simulink model "main_model"  (R2025b)
settings: Solver=VariableStepAuto  StartTime=0.0  StopTime=30  RelTol=1e-3
undefined symbols (not defined in the file or in its folder): A, a, B, C, c, flow_coeff, H, R, W
settings Model: Creator=janek  LastModifiedBy=janek

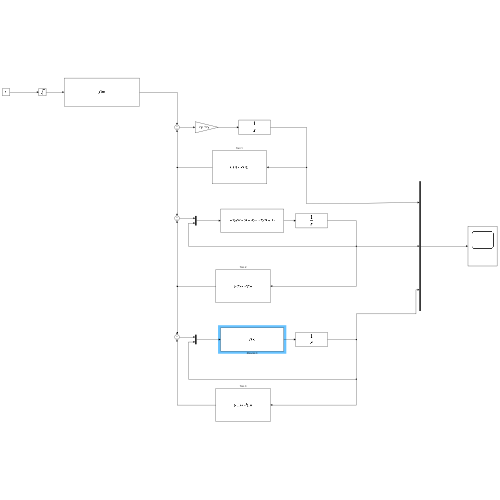
[thumbnail: Simulink's stored preview of the top-level diagram]
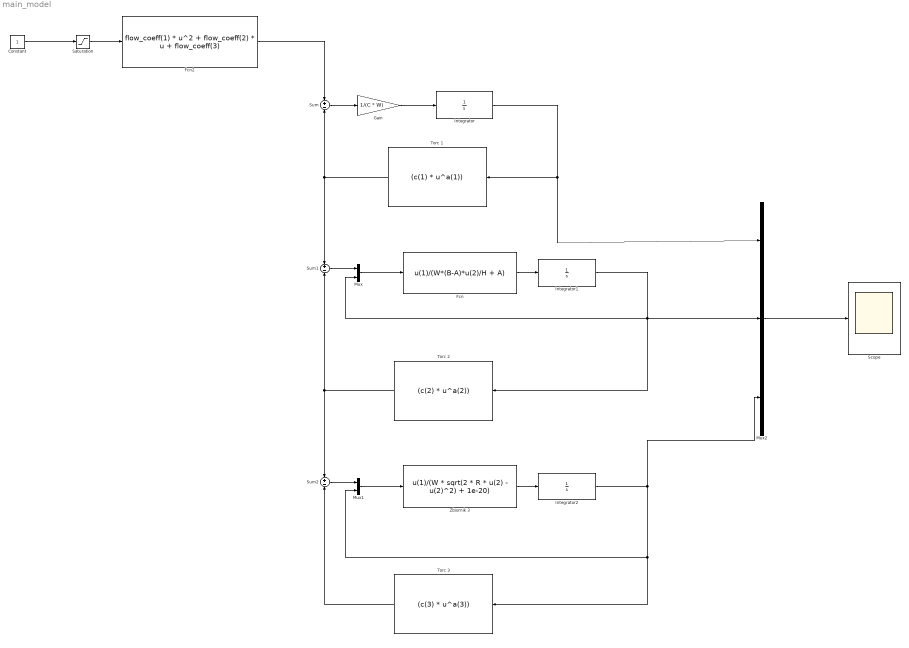
== system main_model ==
  Constant : Constant
  Fcn : Fcn  Expr=u(1)/(W*(B-A)*u(2)/H + A)
  Fcn2 : Fcn  Expr=flow_coeff(1) * u^2 + flow_coeff(2) * u + flow_coeff(3)
  Gain : Gain  Gain=1/(C * W)
  Integrator : Integrator
  Integrator1 : Integrator
  Integrator2 : Integrator
  Mux : Mux  Inputs=2
  Mux1 : Mux  Inputs=2
  Mux2 : Mux  Inputs=3
  Saturation : Saturate  UpperLimit=1  LowerLimit=0.53
  Scope : Scope
      settings: ActiveDisplayYMinimum=-228.8305116738498  ActiveDisplayYMaximum=137.59972861742904
  Sum : Sum  Inputs=+|-
  Sum1 : Sum  Inputs=+|-
  Sum2 : Sum  Inputs=+|-
  Torc 1 : Fcn  Expr=(c(1) * u^a(1))
  Torc 2 : Fcn  Expr=(c(2) * u^a(2))
  Torc 3 : Fcn  Expr=(c(3) * u^a(3))
  Zbiornik 3 : Fcn  Expr=u(1)/(W * sqrt(2 * R * u(2) - u(2)^2) + 1e-20)
  wires:
  Integrator/1 -> Mux2/1, Torc 1/1
  Gain/1 -> Integrator/1
  Sum/1 -> Gain/1
  Torc 1/1 -> Sum/2, Sum1/1
  Sum1/1 -> Mux/1
  Integrator1/1 -> Mux/2, Torc 2/1, Mux2/2
  Fcn/1 -> Integrator1/1
  Mux/1 -> Fcn/1
  Sum2/1 -> Mux1/1
  Torc 3/1 -> Sum2/2
  Torc 2/1 -> Sum2/1, Sum1/2
  Integrator2/1 -> Mux1/2, Torc 3/1, Mux2/3
  Zbiornik 3/1 -> Integrator2/1
  Mux1/1 -> Zbiornik 3/1
  Saturation/1 -> Fcn2/1
  Constant/1 -> Saturation/1
  Mux2/1 -> Scope/1
  Fcn2/1 -> Sum/1
